simulink model "Translationalsim"  (R2023a)
settings: Solver=FixedStepAuto  StartTime=0.0  StopTime=tf  FixedStep=tstep  RelTol=1e-3  EnableMultiTasking=on
values from neighbouring files (symbols this model uses):
  C = [1 0 0 0 0 0;     0 1 0 0 0 0;     0 0 1 0 0 0]    [Attitude.m]    (also in Translational.m = eye(6); UpdatedAttitude.m = [1 0 0 0 0 0;      0 1 0 0 0 0;      0 0 1 0 0 0])
  Cc = [1 0 0 0 0 0;     0 1 0 0 0 0;     0 0 1 0 0 0]    [Translational.m]
  k = 55    [ActuatorModel.m]    (also in SysID.m = 11.93; Translational.m = -inv(R)*Bbar'*P)
  L = Pltr*Co'*inv(Ro)    [Attitude.m]    (also in Translational.m = Pltr*C'*inv(Ro))
  ref = [pi/18 pi/32 0]    [Attitude.m]    (also in Translational.m = [0 0 -2]; main.m = [1;1;-2])
  tstep = 0.001    [ActuatorModel.m]    (also in Attitude.m; Translational.m; UpdatedAttitude.m = 0.0001; main.m)
  xi = [0; pi/6; 0; 0; 0; 0]    [Attitude.m]    (also in Translational.m = [0; 0; 0; 0; 0; 0])
libraries: simulink x1
settings Model: Creator=Nathan Dablain  LastModifiedBy=Nathan Dablain

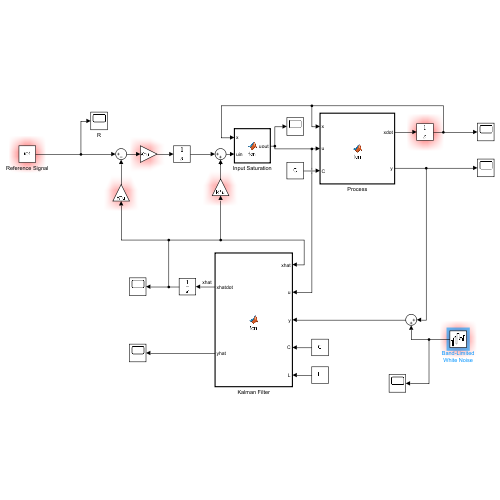
[thumbnail: Simulink's stored preview of the top-level diagram]
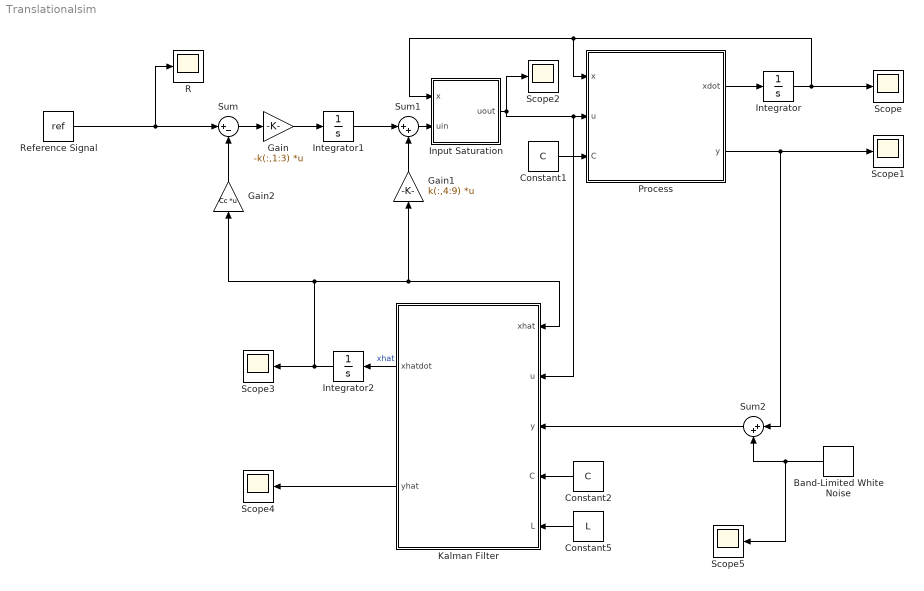
== system Translationalsim ==
  Band-Limited White Noise : simulink/Sources/Band-Limited White Noise  Cov=0.05.*[1e-2 1e-2 1e-2 1e-3 1e-3 1e-3]'  Ts=tstep  seed=[23341]
  Constant1 : Constant  Value=C
  Constant2 : Constant  Value=C
  Constant5 : Constant  Value=L
  Gain : Gain  Gain=-k(:,1:3)  Multiplication=Matrix(K*u)
  Gain1 : Gain  Gain=k(:,4:9)  Multiplication=Matrix(K*u)
  Gain2 : Gain  Gain=Cc  Multiplication=Matrix(K*u)
  Input Saturation : MATLAB Function  TreatAsAtomicUnit=on
  Integrator : Integrator  InitialCondition=xi
  Integrator1 : Integrator  InitialCondition=zeros(4,1)
  Integrator2 : Integrator  InitialCondition=zeros(6,1)
  Kalman Filter : MATLAB Function  TreatAsAtomicUnit=on
  Process : MATLAB Function  TreatAsAtomicUnit=on
  R : Scope
  Reference Signal : Constant  Value=ref
  Scope{,1..5} (6 alike) : Scope
  Sum : Sum  Inputs=|+-
  Sum1 : Sum  Inputs=|++
  Sum2 : Sum  Inputs=|++
  wires:
  Process/1(xdot) -> Integrator/1
  Integrator/1 -> Input Saturation/1(x), Process/1(x), Scope/1
  Process/2(y) -> Sum2/1, Scope1/1
  Constant1/1 -> Process/3(C)
  Integrator1/1 -> Sum1/1
  Sum/1 -> Gain/1
  Gain1/1 -> Sum1/2
  Reference Signal/1 -> R/1, Sum/1
  Sum1/1 -> Input Saturation/2(uin)
  Input Saturation/1(uout) -> Kalman Filter/2(u), Process/2(u), Scope2/1
  Kalman Filter/1(xhatdot) -> Integrator2/1  "xhat"
  Integrator2/1 -> Kalman Filter/1(xhat), Gain1/1, Gain2/1, Scope3/1
  Gain/1 -> Integrator1/1
  Constant2/1 -> Kalman Filter/4(C)
  Constant5/1 -> Kalman Filter/5(L)
  Gain2/1 -> Sum/2
  Band-Limited White Noise/1 -> Scope5/1, Sum2/2
  Kalman Filter/2(yhat) -> Scope4/1
  Sum2/1 -> Kalman Filter/3(y)

== matlab function Translationalsim/Process ==
  data: x input; xdot output; u input; y output; C input
function [xdot,y] = fcn(x,u,C)
m = 2.25;
g = 9.79;

K = 6000; % Ground stiffness (N/m)
c = 200; % Ground damping (N/m/s)
if x(3) >= 0
    Fr = [c*x(4);c*x(5);K*x(3) + c*x(6)]; % Ground reaction force
else
    Fr = zeros(3,1);
end

phi = u(2);
theta = u(3);
psi = u(4);

xdot = [[cos(theta)*cos(psi)  sin(phi)*sin(theta)*cos(psi) - cos(phi)*sin(psi) cos(phi)*sin(theta)*cos(psi)+sin(phi)*sin(psi);... 
    cos(theta)*sin(psi)  sin(phi)*sin(theta)*sin(psi)+cos(phi)*cos(psi) cos(phi)*sin(theta)*sin(psi)-sin(phi)*cos(psi);... 
    -sin(theta) sin(phi)*cos(theta) cos(phi)*cos(theta)]*x(4:6);...
    -g*sin(theta) - Fr(1)/m;...
    g*cos(theta)*sin(phi) - Fr(2)/m;...
    -u(1)/m-Fr(3)/m+g*cos(theta)*cos(phi)];
y = C*x;
end

== matlab function Translationalsim/Input Saturation ==
  data: x input; uin input; uout output
function uout = fcn(x,uin)
uout = uin;
max_ang = 20*pi/180; % rad
max_thrust = 30; % N
if uin(1)> max_thrust
    uout(1) = max_thrust;
elseif uin(1)<0
    uout(1) = 0;
end
for i = 2:4
    if x(3)>=-0.01
        uout(i) = 0;
    elseif uin(i) > max_ang
        uout(i) = max_ang;
    elseif uin(i) < -max_ang
        uout(i) = -max_ang;
    end
end
end

== matlab function Translationalsim/Kalman Filter ==
  data: xhat input; u input; y input; C input; xhatdot output; L input; yhat output
function [xhatdot,yhat]  = fcn(xhat, u, y, C, L)
m = 2.5;
g = 9.81;

K = 5000; % Ground stiffness (N/m)
c = 150; % Ground damping (N/m/s)
if xhat(3) >= 0
    Fr = [c*xhat(4);c*xhat(5);K*xhat(3) + c*xhat(6)]; % Ground reaction force
else
    Fr = zeros(3,1);
end

phi = u(2);
theta = u(3);
psi = u(4);
yhat = C*xhat;
xhatdot = [[cos(theta)*cos(psi)  sin(phi)*sin(theta)*cos(psi) - cos(phi)*sin(psi) cos(phi)*sin(theta)*cos(psi)+sin(phi)*sin(psi);... 
    cos(theta)*sin(psi)  sin(phi)*sin(theta)*sin(psi)+cos(phi)*cos(psi) cos(phi)*sin(theta)*sin(psi)-sin(phi)*cos(psi);... 
    -sin(theta) sin(phi)*cos(theta) cos(phi)*cos(theta)]*xhat(4:6);...
    -g*sin(theta) - Fr(1)/m;...
    g*cos(theta)*sin(phi) - Fr(2)/m;...
    -u(1)/m-Fr(3)/m+g*cos(theta)*cos(phi)] + L*(y-yhat);
end
